simulink model "model3"  (R2024b)
settings: Solver=VariableStepAuto  StartTime=0.0  StopTime=2  MaxStep=1e-3  RelTol=1e-3
settings Model: Creator=mehmetcanevi  LastModifiedBy=mehmetcanevi

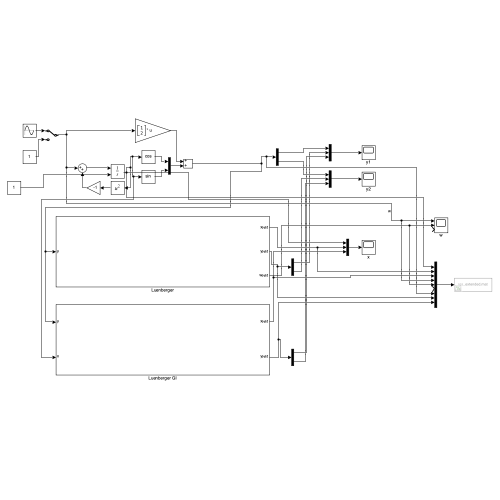
[thumbnail: Simulink's stored preview of the top-level diagram]
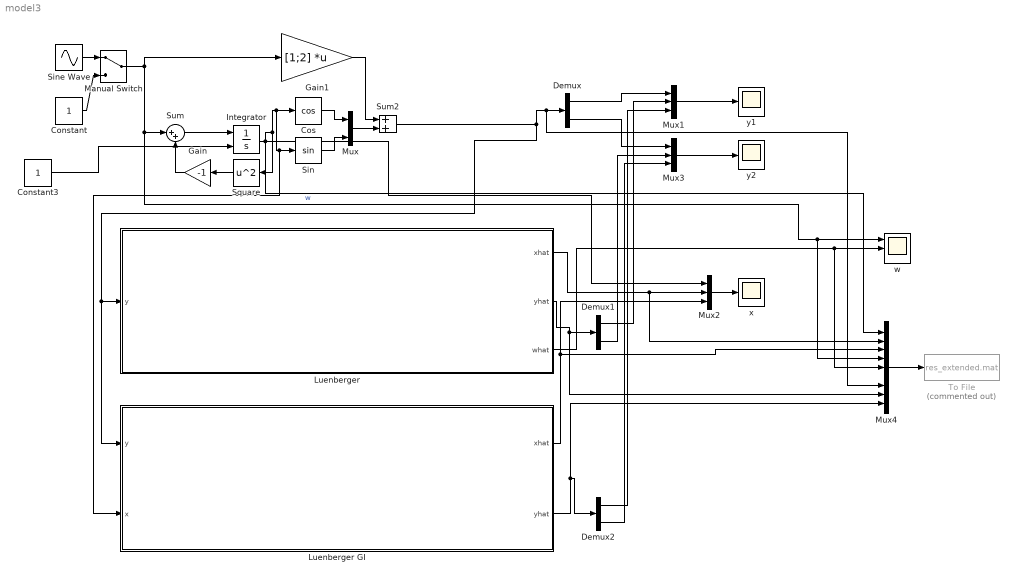
== system model3 ==
  Constant : Constant
  Constant3 : Constant
  Cos : Trigonometry  Operator=cos
  Demux : Demux  Outputs=2
  Demux1 : Demux  Outputs=2
  Demux2 : Demux  Outputs=2
  Gain : Gain  Gain=-1
  Gain1 : Gain  Gain=[1;2]  Multiplication=Matrix(K*u)
  Integrator : Integrator  InitialConditionSource=external
  Luenberger : Subsystem
  Luenberger GI : Subsystem
  Manual Switch : ManualSwitch
  Mux : Mux  Inputs=2
  Mux1 : Mux  Inputs=3
  Mux2 : Mux  Inputs=3
  Mux3 : Mux  Inputs=3
  Mux4 : Mux  Inputs=9
  Sin : Trigonometry
  Sine Wave : Sin  Frequency=10  SampleTime=0
  Square : Math  Operator=square
  Sum : Sum  Inputs=|++
  Sum2 : Sum
  To File : ToFile  Commented=on  Filename=res_extended.mat  MatrixName=data
  w : Scope  NumInputPorts=3
  x : Scope
  y1 : Scope
  y2 : Scope
  wires:
  Integrator/1 -> Mux4/1, Square/1, Luenberger GI/2(x), Sin/1, Cos/1, Mux2/1
  Sum/1 -> Integrator/1
  Cos/1 -> Mux/1
  Square/1 -> Gain/1
  Gain/1 -> Sum/2
  Constant3/1 -> Integrator/2
  Sin/1 -> Mux/2
  Mux/1 -> Sum2/2
  Manual Switch/1 -> Mux4/4, w/1, Sum/1, Gain1/1  "w"
  Gain1/1 -> Sum2/1
  Sum2/1 -> Mux4/7, Demux/1, Luenberger GI/1(y), Luenberger/1(y)
  Mux2/1 -> x/1
  Luenberger/1(xhat) -> Mux4/2, Mux2/2
  Luenberger GI/1(xhat) -> Mux4/3, Mux2/3
  Demux/1 -> Mux1/1
  Mux1/1 -> y1/1
  Mux3/1 -> y2/1
  Demux/2 -> Mux3/1
  Luenberger/2(yhat) -> Mux4/8, Demux1/1
  Demux1/1 -> Mux1/2
  Demux1/2 -> Mux3/2
  Luenberger GI/2(yhat) -> Mux4/9, Demux2/1
  Demux2/1 -> Mux1/3
  Demux2/2 -> Mux3/3
  Sine Wave/1 -> Manual Switch/1
  Constant/1 -> Manual Switch/2
  Mux4/1 -> To File/1
  Luenberger/3(what) -> Mux4/5, w/2

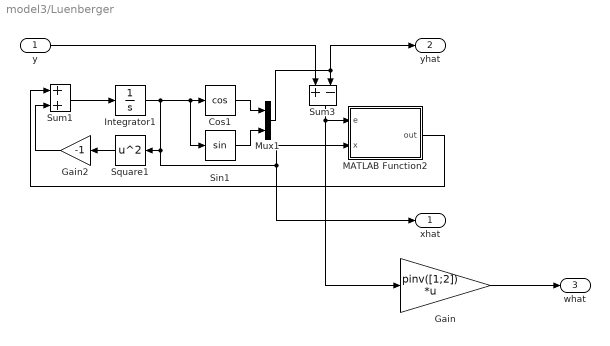
== system model3/Luenberger ==
  y : Inport
  Cos1 : Trigonometry  Operator=cos
  Gain : Gain  Gain=pinv([1;2])  Multiplication=Matrix(K*u)
  Gain2 : Gain  Gain=-1
  Integrator1 : Integrator
  MATLAB Function2 : MATLAB Function  TreatAsAtomicUnit=on
  Mux1 : Mux  Inputs=2
  Sin1 : Trigonometry
  Square1 : Math  Operator=square
  Sum1 : Sum
  Sum3 : Sum  Inputs=+-
  xhat : Outport
  yhat : Outport  Port=2
  what : Outport  Port=3
  wires:
  Sin1/1 -> Mux1/2
  Mux1/1 -> yhat/1, Sum3/2
  Integrator1/1 -> Sin1/1, Cos1/1, MATLAB Function2/2(x), xhat/1, Square1/1
  Cos1/1 -> Mux1/1
  Sum3/1 -> Gain/1, MATLAB Function2/1(e)
  MATLAB Function2/1(out) -> Sum1/1
  Square1/1 -> Gain2/1
  Sum1/1 -> Integrator1/1
  Gain2/1 -> Sum1/2
  y/1 -> Sum3/1
  Gain/1 -> what/1

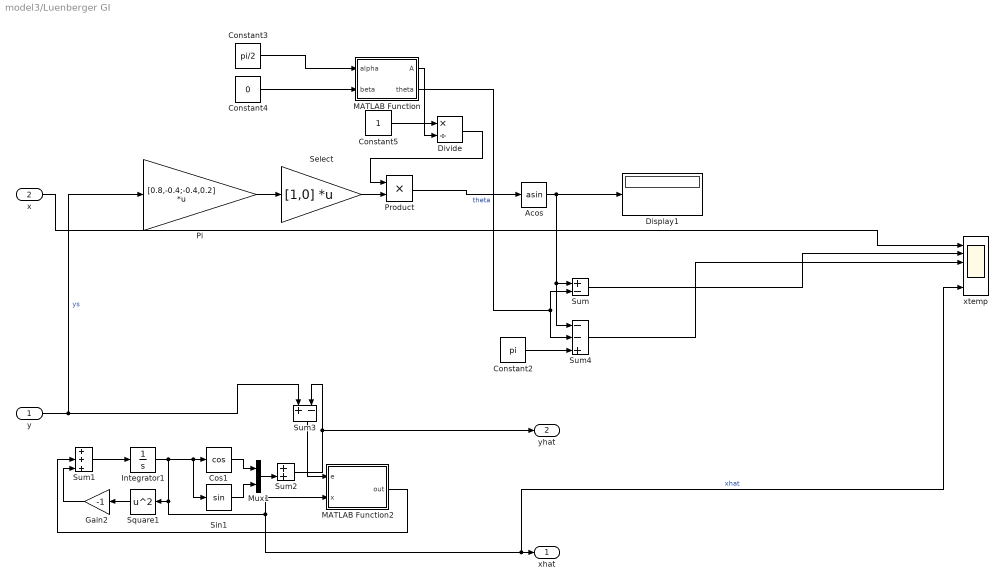
== system model3/Luenberger GI ==
  y : Inport
  x : Inport  Port=2
  Acos : Trigonometry  Operator=asin
  Constant2 : Constant  Value=pi
  Constant3 : Constant  Value=pi/2
  Constant4 : Constant  Value=0
  Constant5 : Constant
  Cos1 : Trigonometry  Operator=cos
  Display1 : Display
  Divide : Product  Inputs=*/
  Gain2 : Gain  Gain=-1
  Integrator1 : Integrator
  MATLAB Function : MATLAB Function  TreatAsAtomicUnit=on
  MATLAB Function2 : MATLAB Function  TreatAsAtomicUnit=on
  Mux1 : Mux  Inputs=2
  Pi : Gain  Gain=[0.8,-0.4;-0.4,0.2]  Multiplication=Matrix(K*u)
  Product : Product
  Select : Gain  Gain=[1,0]  Multiplication=Matrix(K*u)
  Sin1 : Trigonometry
  Square1 : Math  Operator=square
  Sum : Sum  Inputs=+-
  Sum1 : Sum  Inputs=+++
  Sum2 : Sum
  Sum3 : Sum  Inputs=+-
  Sum4 : Sum  Inputs=--+
  xtemp : Scope  NumInputPorts=6
  xhat : Outport
  yhat : Outport  Port=2
  wires:
  Gain2/1 -> Sum1/3
  Sum1/1 -> Integrator1/1
  Square1/1 -> Gain2/1
  MATLAB Function2/1(out) -> Sum1/2
  Sum3/1 -> MATLAB Function2/1(e)
  Cos1/1 -> Mux1/1
  Integrator1/1 -> Square1/1, xtemp/6, xhat/1, MATLAB Function2/2(x), Cos1/1, Sin1/1  "xhat"
  Sum2/1 -> Sum3/2, yhat/1
  Sin1/1 -> Mux1/2
  y/1 -> Pi/1, Sum3/1  "ys"
  Mux1/1 -> Sum2/2
  Pi/1 -> Select/1
  Select/1 -> Product/2
  Product/1 -> Acos/1
  Acos/1 -> Display1/1, Sum4/1, Sum/1
  x/1 -> xtemp/1
  MATLAB Function/2(theta) -> Sum/2, Sum4/2  "theta"
  Sum/1 -> xtemp/2
  Constant2/1 -> Sum4/3
  Sum4/1 -> xtemp/3
  Constant3/1 -> MATLAB Function/1(alpha)
  Constant4/1 -> MATLAB Function/2(beta)
  Constant5/1 -> Divide/1
  MATLAB Function/1(A) -> Divide/2
  Divide/1 -> Product/1

== matlab function model3/Luenberger/MATLAB Function2 ==
  data: e input; out output; x input
function out= fcn(e,x)
lambda=-10;
l2=(lambda+2*x-sin(x))/(-2*sin(x)-cos(x));
l1=1-2*l2;
out=[l1,l2]*e;
end

== matlab function model3/Luenberger GI/MATLAB Function2 ==
  data: e input; out output; x input
function out= fcn(e,x)
if -2*sin(x)-cos(x)>0
    lambda=-10;
    l2=(lambda+2*x-sin(x))/(-2*sin(x)-cos(x));
    l1=1-2*l2;
    out=[l1,l2]*e;
else
    lambda=-10;
    l2=(lambda+2*x-sin(x))/(-2*sin(x)-cos(x)+0.1);
    l1=1-2*l2;
    out=[l1,l2]*e;
end

end

== matlab function model3/Luenberger GI/MATLAB Function ==
  data: alpha input; A output; beta input; theta output
function [A,theta] = fcn(alpha,beta)

Pival=[0.8,-0.4;-0.4,0.2];
yv=Pival(1,1)*sin(alpha)+Pival(1,2)*sin(beta);
xv=Pival(1,1)*cos(alpha)+Pival(1,2)*cos(beta);
A=sqrt(xv^2+yv^2);
theta=atan2(yv,xv);
end
